simulink model "sub33isOK"  (Simulink 7.2)
settings: Solver=ode45  StartTime=0.0  StopTime=10.0  RelTol=1e-3
undefined symbols (not defined in the file): ln
settings Model: Creator=hp  LastModifiedBy=hp

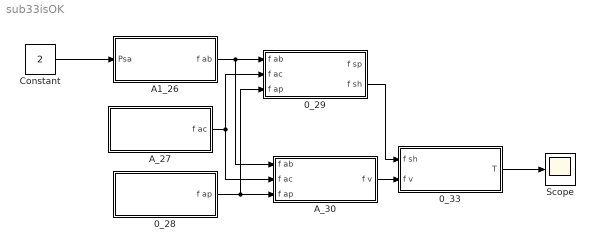
== system sub33isOK ==
  0_28 : Subsystem
  0_29 : Subsystem
  0_33 : Subsystem
  A1_26 : Subsystem
  A_27 : Subsystem
  A_30 : Subsystem
  Constant : Constant  Value=2  OutDataType=sfix(16)  OutScaling=2^0
  Scope : Scope
  wires:
  0_28/1(f ap) -> A_30/3(f ap), 0_29/3(f ap)
  A_27/1(f ac) -> A_30/2(f ac), 0_29/2(f ac)
  A1_26/1(f ab) -> A_30/1(f ab), 0_29/1(f ab)
  Constant/1 -> A1_26/1(Psa)
  A_30/1(f v) -> 0_33/2(f v)
  0_29/2(f sh) -> 0_33/1(f sh)
  0_33/1(T) -> Scope/1

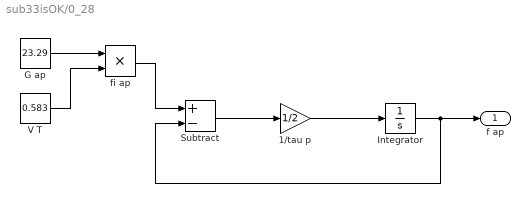
== system sub33isOK/0_28 ==
  1/tau p : Gain  Gain=1/2  ParameterDataType=sfix(16)  ParameterScaling=2^0  OutDataType=sfix(16)  OutScaling=2^0
  G ap : Constant  Value=23.29  OutDataType=sfix(16)  OutScaling=2^0
  Integrator : Integrator
  Subtract : Sum  Inputs=+-  OutDataType=sfix(16)  OutScaling=2^-10
  V T : Constant  Value=0.583  OutDataType=sfix(16)  OutScaling=2^0
  fi ap : Product  OutDataType=sfix(16)  OutScaling=2^0  RndMeth=Zero
  f ap : Outport  OutDataType=sfix(16)  OutScaling=2^0
  wires:
  Integrator/1 -> f ap/1, Subtract/2
  1/tau p/1 -> Integrator/1
  Subtract/1 -> 1/tau p/1
  fi ap/1 -> Subtract/1
  G ap/1 -> fi ap/1
  V T/1 -> fi ap/2

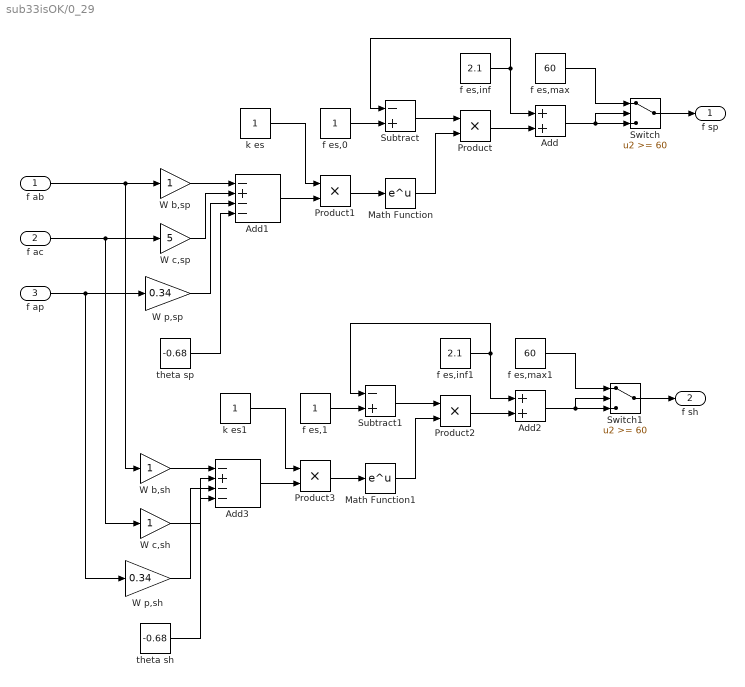
== system sub33isOK/0_29 ==
  f ab : Inport  OutDataType=sfix(16)  OutScaling=2^0
  f ac : Inport  Port=2  OutDataType=sfix(16)  OutScaling=2^0
  f ap : Inport  Port=3  OutDataType=sfix(16)  OutScaling=2^0
  Add : Sum  OutDataType=sfix(16)  OutScaling=2^-10
  Add1 : Sum  Inputs=-+--  OutDataType=sfix(16)  OutScaling=2^-10
  Add2 : Sum  OutDataType=sfix(16)  OutScaling=2^-10
  Add3 : Sum  Inputs=-+--  OutDataType=sfix(16)  OutScaling=2^-10
  Math Function : Math  OutDataType=sfix(16)  OutScaling=2^0  SaturateOnIntegerOverflow=on
  Math Function1 : Math  OutDataType=sfix(16)  OutScaling=2^0  SaturateOnIntegerOverflow=on
  Product{,1..3} (4 alike) : Product  OutDataType=sfix(16)  OutScaling=2^0  RndMeth=Zero
  Subtract : Sum  Inputs=-+  OutDataType=sfix(16)  OutScaling=2^-10
  Subtract1 : Sum  Inputs=-+  OutDataType=sfix(16)  OutScaling=2^-10
  Switch : Switch  Threshold=60  OutDataType=sfix(16)  OutScaling=2^0
  Switch1 : Switch  Threshold=60  OutDataType=sfix(16)  OutScaling=2^0
  W b,sh : Gain  ParameterDataType=sfix(16)  ParameterScaling=2^0  OutDataType=sfix(16)  OutScaling=2^0
  W b,sp : Gain  ParameterDataType=sfix(16)  ParameterScaling=2^0  OutDataType=sfix(16)  OutScaling=2^0
  W c,sh : Gain  ParameterDataType=sfix(16)  ParameterScaling=2^0  OutDataType=sfix(16)  OutScaling=2^0
  W c,sp : Gain  Gain=5  ParameterDataType=sfix(16)  ParameterScaling=2^0  OutDataType=sfix(16)  OutScaling=2^0
  W p,sh : Gain  Gain=0.34  ParameterDataType=sfix(16)  ParameterScaling=2^0  OutDataType=sfix(16)  OutScaling=2^0
  W p,sp : Gain  Gain=0.34  ParameterDataType=sfix(16)  ParameterScaling=2^0  OutDataType=sfix(16)  OutScaling=2^0
  f es,0 : Constant  OutDataType=sfix(16)  OutScaling=2^0
  f es,1 : Constant  OutDataType=sfix(16)  OutScaling=2^0
  f es,inf : Constant  Value=2.1  OutDataType=sfix(16)  OutScaling=2^0
  f es,inf1 : Constant  Value=2.1  OutDataType=sfix(16)  OutScaling=2^0
  f es,max : Constant  Value=60  OutDataType=sfix(16)  OutScaling=2^0
  f es,max1 : Constant  Value=60  OutDataType=sfix(16)  OutScaling=2^0
  k es : Constant  OutDataType=sfix(16)  OutScaling=2^0
  k es1 : Constant  OutDataType=sfix(16)  OutScaling=2^0
  theta sh : Constant  Value=-0.68  OutDataType=sfix(16)  OutScaling=2^0
  theta sp : Constant  Value=-0.68  OutDataType=sfix(16)  OutScaling=2^0
  f sp : Outport  OutDataType=sfix(16)  OutScaling=2^0
  f sh : Outport  Port=2  OutDataType=sfix(16)  OutScaling=2^0
  wires:
  Add3/1 -> Product3/2
  theta sh/1 -> Add3/4
  W p,sh/1 -> Add3/3
  W c,sh/1 -> Add3/2
  W b,sh/1 -> Add3/1
  k es1/1 -> Product3/1
  Product3/1 -> Math Function1/1
  Math Function1/1 -> Product2/2
  f es,1/1 -> Subtract1/2
  Subtract1/1 -> Product2/1
  Product2/1 -> Add2/2
  f es,inf1/1 -> Subtract1/1, Add2/1
  Add2/1 -> Switch1/3, Switch1/2
  Switch1/1 -> f sh/1
  f es,max1/1 -> Switch1/1
  Add1/1 -> Product1/2
  theta sp/1 -> Add1/4
  W p,sp/1 -> Add1/3
  f ap/1 -> W p,sh/1, W p,sp/1
  f ac/1 -> W c,sh/1, W c,sp/1
  W c,sp/1 -> Add1/2
  f ab/1 -> W b,sh/1, W b,sp/1
  W b,sp/1 -> Add1/1
  k es/1 -> Product1/1
  Product1/1 -> Math Function/1
  Math Function/1 -> Product/2
  f es,0/1 -> Subtract/2
  Subtract/1 -> Product/1
  Product/1 -> Add/2
  f es,inf/1 -> Subtract/1, Add/1
  Add/1 -> Switch/3, Switch/2
  Switch/1 -> f sp/1
  f es,max/1 -> Switch/1

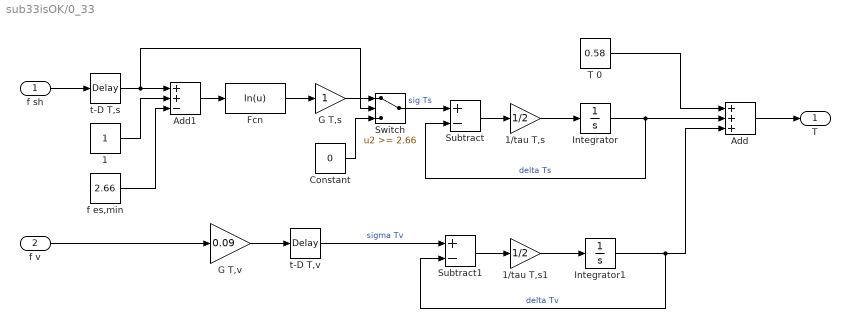
== system sub33isOK/0_33 ==
  f sh : Inport  OutDataType=sfix(16)  OutScaling=2^0
  f v : Inport  Port=2  OutDataType=sfix(16)  OutScaling=2^0
  1 : Constant  OutDataType=sfix(16)  OutScaling=2^0
  1/tau T,s : Gain  Gain=1/2  ParameterDataType=sfix(16)  ParameterScaling=2^0  OutDataType=sfix(16)  OutScaling=2^0
  1/tau T,s1 : Gain  Gain=1/2  ParameterDataType=sfix(16)  ParameterScaling=2^0  OutDataType=sfix(16)  OutScaling=2^0
  Add : Sum  Inputs=+++  OutDataType=sfix(16)  OutScaling=2^-10
  Add1 : Sum  Inputs=++-  OutDataType=sfix(16)  OutScaling=2^-10
  Constant : Constant  Value=0  OutDataType=sfix(16)  OutScaling=2^0
  Fcn : Fcn  Expr=ln(u)
  G T,s : Gain  ParameterDataType=sfix(16)  ParameterScaling=2^0  OutDataType=sfix(16)  OutScaling=2^0
  G T,v : Gain  Gain=0.09  ParameterDataType=sfix(16)  ParameterScaling=2^0  OutDataType=sfix(16)  OutScaling=2^0
  Integrator : Integrator
  Integrator1 : Integrator
  Subtract : Sum  Inputs=+-  OutDataType=sfix(16)  OutScaling=2^-10
  Subtract1 : Sum  Inputs=+-  OutDataType=sfix(16)  OutScaling=2^-10
  Switch : Switch  Threshold=2.66  OutDataType=sfix(16)  OutScaling=2^0
  T 0 : Constant  Value=0.58  OutDataType=sfix(16)  OutScaling=2^0
  f es,min : Constant  Value=2.66  OutDataType=sfix(16)  OutScaling=2^0
  t-D T,s : TransportDelay  DelayTime=2
  t-D T,v : TransportDelay  DelayTime=0.2
  T : Outport  OutDataType=sfix(16)  OutScaling=2^0
  wires:
  Switch/1 -> Subtract/1  "sig Ts"
  Constant/1 -> Switch/3
  G T,s/1 -> Switch/1
  Add1/1 -> Fcn/1
  f es,min/1 -> Add1/3
  1/1 -> Add1/2
  t-D T,s/1 -> Add1/1, Switch/2
  f sh/1 -> t-D T,s/1
  Fcn/1 -> G T,s/1
  t-D T,v/1 -> Subtract1/1  "sigma Tv"
  G T,v/1 -> t-D T,v/1
  f v/1 -> G T,v/1
  T 0/1 -> Add/1
  Add/1 -> T/1
  Subtract1/1 -> 1/tau T,s1/1
  Integrator/1 -> Add/2, Subtract/2  "delta Ts"
  Subtract/1 -> 1/tau T,s/1
  1/tau T,s/1 -> Integrator/1
  1/tau T,s1/1 -> Integrator1/1
  Integrator1/1 -> Subtract1/2, Add/3  "delta Tv"

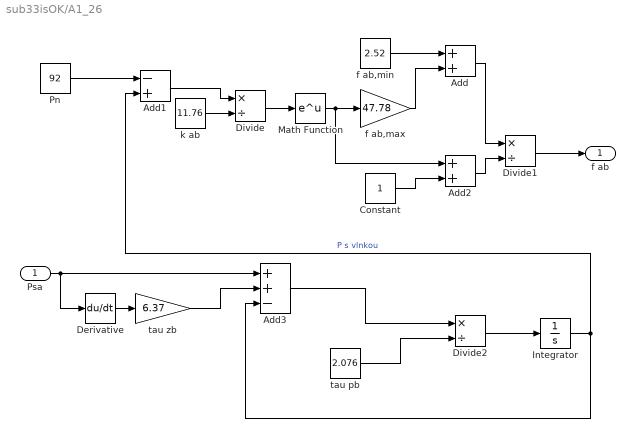
== system sub33isOK/A1_26 ==
  Psa : Inport  OutDataType=sfix(16)  OutScaling=2^0
  Add : Sum  OutDataType=sfix(16)  OutScaling=2^-10
  Add1 : Sum  Inputs=-+  OutDataType=sfix(16)  OutScaling=2^-10
  Add2 : Sum  OutDataType=sfix(16)  OutScaling=2^-10
  Add3 : Sum  Inputs=++-  OutDataType=sfix(16)  OutScaling=2^-10
  Constant : Constant  OutDataType=sfix(16)  OutScaling=2^0
  Derivative : Derivative
  Divide : Product  Inputs=*/  OutDataType=sfix(16)  OutScaling=2^-10
  Divide1 : Product  Inputs=*/  OutDataType=sfix(16)  OutScaling=2^-10
  Divide2 : Product  Inputs=*/  OutDataType=sfix(16)  OutScaling=2^-10
  Integrator : Integrator
  Math Function : Math  OutDataType=sfix(16)  OutScaling=2^0  SaturateOnIntegerOverflow=on
  Pn : Constant  Value=92  OutDataType=sfix(16)  OutScaling=2^0
  f ab,max : Gain  Gain=47.78  ParameterDataType=sfix(16)  ParameterScaling=2^0  OutDataType=sfix(16)  OutScaling=2^0
  f ab,min : Constant  Value=2.52  OutDataType=sfix(16)  OutScaling=2^0
  k ab : Constant  Value=11.76  OutDataType=sfix(16)  OutScaling=2^0
  tau pb : Constant  Value=2.076  OutDataType=sfix(16)  OutScaling=2^0
  tau zb : Gain  Gain=6.37  ParameterDataType=sfix(16)  ParameterScaling=2^0  OutDataType=sfix(16)  OutScaling=2^0
  f ab : Outport  OutDataType=sfix(16)  OutScaling=2^0
  wires:
  f ab,min/1 -> Add/1
  f ab,max/1 -> Add/2
  Math Function/1 -> f ab,max/1, Add2/1
  Divide/1 -> Math Function/1
  k ab/1 -> Divide/2
  Add1/1 -> Divide/1
  Pn/1 -> Add1/1
  Add/1 -> Divide1/1
  Divide1/1 -> f ab/1
  Add2/1 -> Divide1/2
  Constant/1 -> Add2/2
  tau pb/1 -> Divide2/2
  Psa/1 -> Add3/1, Derivative/1
  Derivative/1 -> tau zb/1
  tau zb/1 -> Add3/2
  Add3/1 -> Divide2/1
  Divide2/1 -> Integrator/1
  Integrator/1 -> Add3/3, Add1/2  "P s vlnkou"

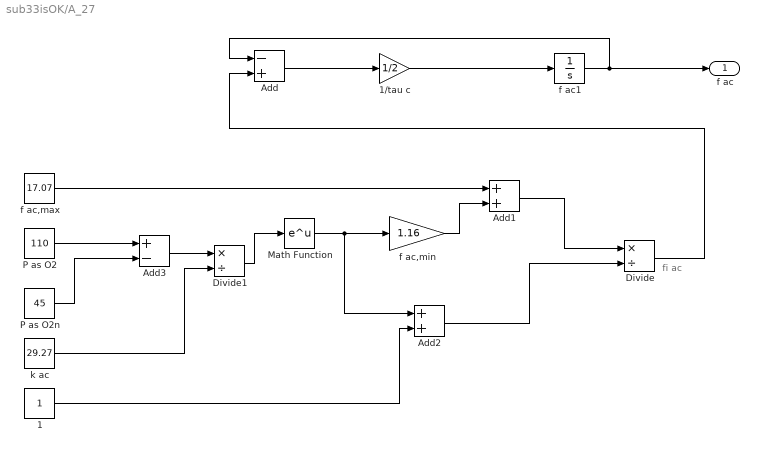
== system sub33isOK/A_27 ==
  note: fi ac
  1 : Constant  OutDataType=sfix(16)  OutScaling=2^0
  1/tau c : Gain  Gain=1/2  ParameterDataType=sfix(16)  ParameterScaling=2^0  OutDataType=sfix(16)  OutScaling=2^0
  Add : Sum  Inputs=-+  OutDataType=sfix(16)  OutScaling=2^-10
  Add1 : Sum  OutDataType=sfix(16)  OutScaling=2^-10
  Add2 : Sum  OutDataType=sfix(16)  OutScaling=2^-10
  Add3 : Sum  Inputs=+-  OutDataType=sfix(16)  OutScaling=2^-10
  Divide : Product  Inputs=*/  OutDataType=sfix(16)  OutScaling=2^-10
  Divide1 : Product  Inputs=*/  OutDataType=sfix(16)  OutScaling=2^-10
  Math Function : Math  OutDataType=sfix(16)  OutScaling=2^0  SaturateOnIntegerOverflow=on
  P as O2 : Constant  Value=110  OutDataType=sfix(16)  OutScaling=2^0
  P as O2n : Constant  Value=45  OutDataType=sfix(16)  OutScaling=2^0
  f ac,max : Constant  Value=17.07  OutDataType=sfix(16)  OutScaling=2^0
  f ac,min : Gain  Gain=1.16  ParameterDataType=sfix(16)  ParameterScaling=2^0  OutDataType=sfix(16)  OutScaling=2^0
  f ac1 : Integrator
  k ac : Constant  Value=29.27  OutDataType=sfix(16)  OutScaling=2^0
  f ac : Outport  OutDataType=sfix(16)  OutScaling=2^0
  wires:
  Divide/1 -> Add/2
  P as O2n/1 -> Add3/2
  P as O2/1 -> Add3/1
  Add3/1 -> Divide1/1
  k ac/1 -> Divide1/2
  Divide1/1 -> Math Function/1
  1/1 -> Add2/2
  Add2/1 -> Divide/2
  Add1/1 -> Divide/1
  f ac,min/1 -> Add1/2
  f ac,max/1 -> Add1/1
  Math Function/1 -> Add2/1, f ac,min/1
  1/tau c/1 -> f ac1/1
  Add/1 -> 1/tau c/1
  f ac1/1 -> Add/1, f ac/1

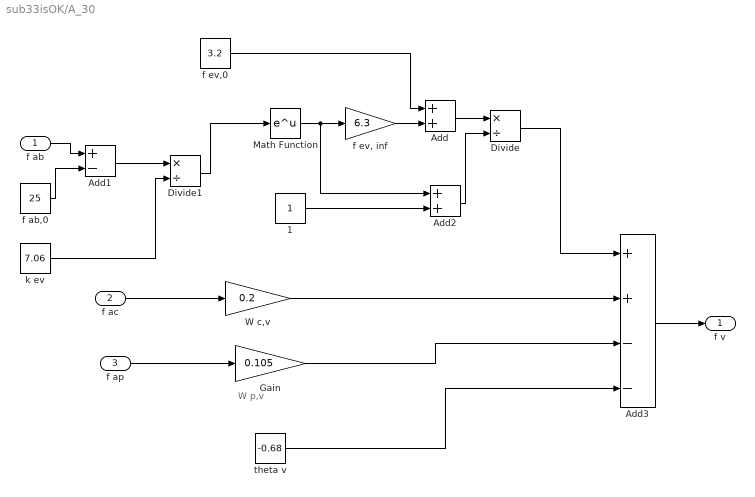
== system sub33isOK/A_30 ==
  note: W p,v
  f ab : Inport  OutDataType=sfix(16)  OutScaling=2^0
  f ac : Inport  Port=2  OutDataType=sfix(16)  OutScaling=2^0
  f ap : Inport  Port=3  OutDataType=sfix(16)  OutScaling=2^0
  1 : Constant  OutDataType=sfix(16)  OutScaling=2^0
  Add : Sum  OutDataType=sfix(16)  OutScaling=2^-10
  Add1 : Sum  Inputs=+-  OutDataType=sfix(16)  OutScaling=2^-10
  Add2 : Sum  OutDataType=sfix(16)  OutScaling=2^-10
  Add3 : Sum  Inputs=++--  OutDataType=sfix(16)  OutScaling=2^-10
  Divide : Product  Inputs=*/  OutDataType=sfix(16)  OutScaling=2^-10
  Divide1 : Product  Inputs=*/  OutDataType=sfix(16)  OutScaling=2^-10
  Gain : Gain  Gain=0.105  ParameterDataType=sfix(16)  ParameterScaling=2^0  OutDataType=sfix(16)  OutScaling=2^0
  Math Function : Math  OutDataType=sfix(16)  OutScaling=2^0  SaturateOnIntegerOverflow=on
  W c,v : Gain  Gain=0.2  ParameterDataType=sfix(16)  ParameterScaling=2^0  OutDataType=sfix(16)  OutScaling=2^0
  f ab,0 : Constant  Value=25  OutDataType=sfix(16)  OutScaling=2^0
  "f ev, inf" : Gain  Gain=6.3  ParameterDataType=sfix(16)  ParameterScaling=2^0  OutDataType=sfix(16)  OutScaling=2^0
  f ev,0 : Constant  Value=3.2  OutDataType=sfix(16)  OutScaling=2^0
  k ev : Constant  Value=7.06  OutDataType=sfix(16)  OutScaling=2^0
  theta v : Constant  Value=-0.68  OutDataType=sfix(16)  OutScaling=2^0
  f v : Outport  OutDataType=sfix(16)  OutScaling=2^0
  wires:
  Add/1 -> Divide/1
  f ev,0/1 -> Add/1
  "f ev, inf"/1 -> Add/2
  Math Function/1 -> "f ev, inf"/1, Add2/1
  f ab/1 -> Add1/1
  f ab,0/1 -> Add1/2
  Add1/1 -> Divide1/1
  Divide1/1 -> Math Function/1
  k ev/1 -> Divide1/2
  Add2/1 -> Divide/2
  1/1 -> Add2/2
  Divide/1 -> Add3/1
  Add3/1 -> f v/1
  W c,v/1 -> Add3/2
  f ac/1 -> W c,v/1
  f ap/1 -> Gain/1
  Gain/1 -> Add3/3
  theta v/1 -> Add3/4
